simulink model "Boundary_Method"  (R2021a)
settings: Solver=VariableStepAuto  StartTime=0.0  StopTime=10.0  RelTol=1e-3
values from neighbouring files (symbols this model uses):
  a = 5.3    [phase_portraits.m]    (also in vs_control_ex2.m = 8)
  b = 1.5    [phase_portraits.m]    (also in vs_control_ex2.m = 15)
  c = 10    [vs_control_ex2.m]
  K = 150    [vs_control_ex2.m]
undefined symbols (not defined in the file or in its folder): b_w, dist, ss_st, yd, ydd
settings Model: Creator=root  LastModifiedBy=root
settings DebuggingCC: MaxConsecutiveZCsMsg=none

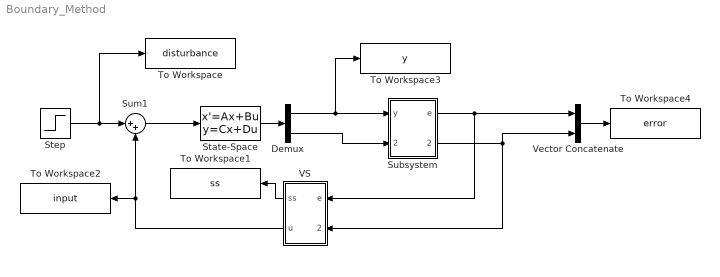
== system Boundary_Method ==
  Demux : Demux  Outputs=2
  State-Space : StateSpace  A=[0 1; -b -a]  B=[0; 1]  C=eye(2)  D=zeros(2, 1)  InitialCondition=[0 0]
  Step : Step  Time=t  After=dist  SampleTime=ss_st
  Subsystem : Subsystem
  Sum1 : Sum  Inputs=|++
  To Workspace : ToWorkspace  VariableName=disturbance  SaveFormat=Timeseries  SampleTime=-1
  To Workspace1 : ToWorkspace  VariableName=ss  SaveFormat=Timeseries  SampleTime=-1
  To Workspace2 : ToWorkspace  VariableName=input  SaveFormat=Timeseries  SampleTime=-1
  To Workspace3 : ToWorkspace  VariableName=y  SaveFormat=Timeseries  SampleTime=-1
  To Workspace4 : ToWorkspace  VariableName=error  SaveFormat=Timeseries  SampleTime=-1
  VS : Subsystem
  Vector Concatenate : Concatenate
  wires:
  Subsystem/2(edot) -> VS/2(edot), Vector Concatenate/2
  Subsystem/1(e) -> VS/1(e), Vector Concatenate/1
  State-Space/1 -> Demux/1
  Vector Concatenate/1 -> To Workspace4/1
  VS/2(u) -> To Workspace2/1, Sum1/2
  Demux/2 -> Subsystem/2(ydot)
  Sum1/1 -> State-Space/1
  Step/1 -> To Workspace/1, Sum1/1
  Demux/1 -> To Workspace3/1, Subsystem/1(y)
  VS/1(ss) -> To Workspace1/1

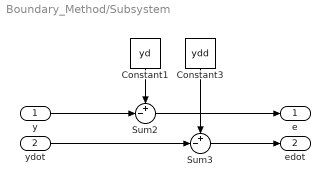
== system Boundary_Method/Subsystem ==
  y : Inport
  ydot : Inport  Port=2
  Constant1 : Constant  Value=yd
  Constant3 : Constant  Value=ydd
  Sum2 : Sum  Inputs=+-|
  Sum3 : Sum  Inputs=+-|
  e : Outport
  edot : Outport  Port=2
  wires:
  Constant1/1 -> Sum2/1
  Sum2/1 -> e/1
  Constant3/1 -> Sum3/1
  Sum3/1 -> edot/1
  ydot/1 -> Sum3/2
  y/1 -> Sum2/2

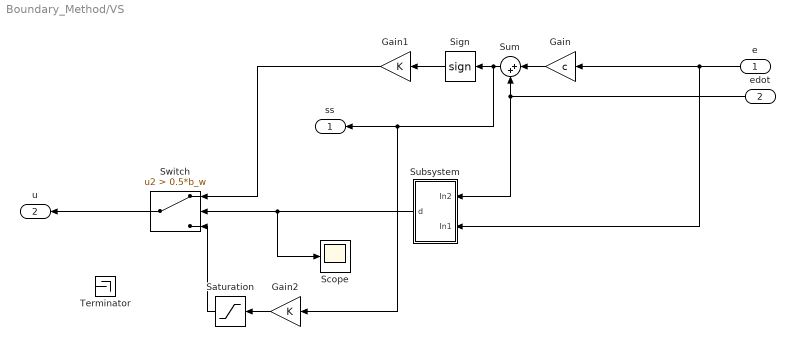
== system Boundary_Method/VS ==
  e : Inport
  edot : Inport  Port=2
  Gain : Gain  Gain=c
  Gain1 : Gain  Gain=K
  Gain2 : Gain  Gain=K
  Saturation : Saturate  UpperLimit=1000  LowerLimit=-1000  ZeroCross=off
  Scope : Scope
  Sign : Signum  ZeroCross=off
  Subsystem : Subsystem
  Sum : Sum  Inputs=|++
  Switch : Switch  Criteria=u2 > Threshold  Threshold=0.5*b_w  ZeroCross=off
  Terminator : Terminator
  ss : Outport
  u : Outport  Port=2
  wires:
  Sign/1 -> Gain1/1
  Gain/1 -> Sum/1
  e/1 -> Subsystem/2(In1), Gain/1
  edot/1 -> Subsystem/1(In2), Sum/2
  Subsystem/1(d) -> Scope/1, Switch/2
  Gain1/1 -> Switch/1
  Switch/1 -> u/1
  Sum/1 -> Gain2/1, ss/1, Sign/1
  Gain2/1 -> Saturation/1
  Saturation/1 -> Switch/3

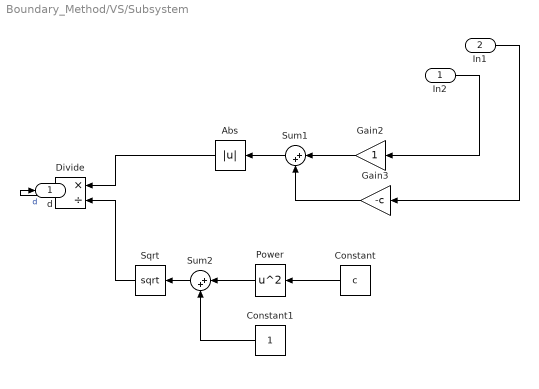
== system Boundary_Method/VS/Subsystem ==
  In2 : Inport
  In1 : Inport  Port=2
  Abs : Abs
  Constant : Constant  Value=c
  Constant1 : Constant
  Divide : Product  Inputs=*/
  Gain2 : Gain
  Gain3 : Gain  Gain=-c
  Power : Math  Operator=square  SaturateOnIntegerOverflow=on
  Sqrt : Sqrt  SaturateOnIntegerOverflow=on
  Sum1 : Sum  Inputs=|++
  Sum2 : Sum  Inputs=|++
  d : Outport
  wires:
  Sqrt/1 -> Divide/2
  Abs/1 -> Divide/1
  Sum1/1 -> Abs/1
  Sum2/1 -> Sqrt/1
  Gain3/1 -> Sum1/2
  Power/1 -> Sum2/1
  In1/1 -> Gain3/1
  Gain2/1 -> Sum1/1
  In2/1 -> Gain2/1
  Constant/1 -> Power/1
  Constant1/1 -> Sum2/2
  Divide/1 -> d/1  "d"
